simulink model "Genearating_MIAC_ZTransform_PLC_Coder_external_Tustin"  (R2018b)
settings: Solver=FixedStepDiscrete  StartTime=0.0  StopTime=30  FixedStep=1  RelTol=1e-3
libraries: simulink x2, slident x2
(part 2 of 2)

== system Genearating_MIAC_ZTransform_PLC_Coder_external_Tustin/Smith_Predictor_MIAC2/System Identification/PT1_Tustin2 ==
  PT1_Input : Inport
  Gain_System : Inport  Port=2
  Time_Constant_System : Inport  Port=3
  Sample_Time : Inport  Port=4
  Reset : Inport  Port=5
  Add : Sum
  Add1 : Sum
  Constant : Constant
  Discrete Transfer Fcn : DiscreteTransferFcn  NumeratorSource=Input port  DenominatorSource=Input port  ExternalReset=Rising  SampleTime=1  a0EqualsOne=on
      settings: InputPortMap=u0,p1,p3,r7
  Divide : Product  Inputs=*/
  Divide1 : Product  Inputs=*/
  Gain : Gain  Gain=2
  Gain1 : Gain  Gain=-1
  Minus : Sum  Inputs=+-
  Multiply : Product
  Mux : Mux  Inputs=2
  Mux1 : Mux  Inputs=2
  PT1_Output : Outport
  wires:
  PT1_Input/1 -> Discrete Transfer Fcn/1
  Mux/1 -> Discrete Transfer Fcn/3
  Sample_Time/1 -> Add1/2, Minus/2, Add/1, Multiply/2
  Mux1/1 -> Discrete Transfer Fcn/2
  Time_Constant_System/1 -> Gain/1
  Discrete Transfer Fcn/1 -> PT1_Output/1
  Gain_System/1 -> Multiply/1
  Multiply/1 -> Divide/1
  Gain/1 -> Add1/1, Minus/1, Add/2
  Add/1 -> Divide/2
  Divide/1 -> Mux1/2, Mux1/1
  Constant/1 -> Mux/1
  Minus/1 -> Divide1/1
  Add1/1 -> Divide1/2
  Divide1/1 -> Gain1/1
  Gain1/1 -> Mux/2
  Reset/1 -> Discrete Transfer Fcn/4
